simulink model "Lab_PMSM_Trial2"  (R2024a)
settings: Solver=VariableStepAuto  StartTime=0.0  StopTime=10  RelTol=1e-3
libraries: spsabctoAlphaBetaZeroLib x2
settings Model: Creator=VICTUS  LastModifiedBy=VICTUS

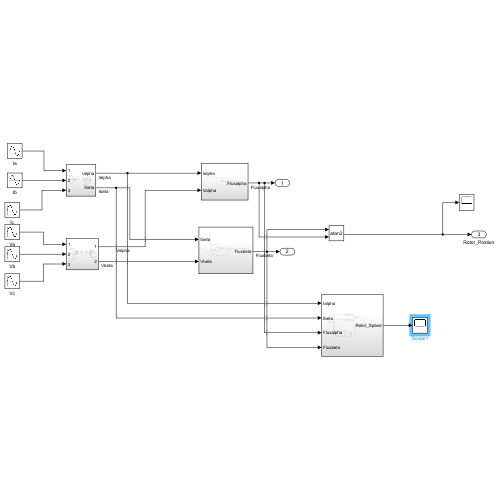
[thumbnail: Simulink's stored preview of the top-level diagram]
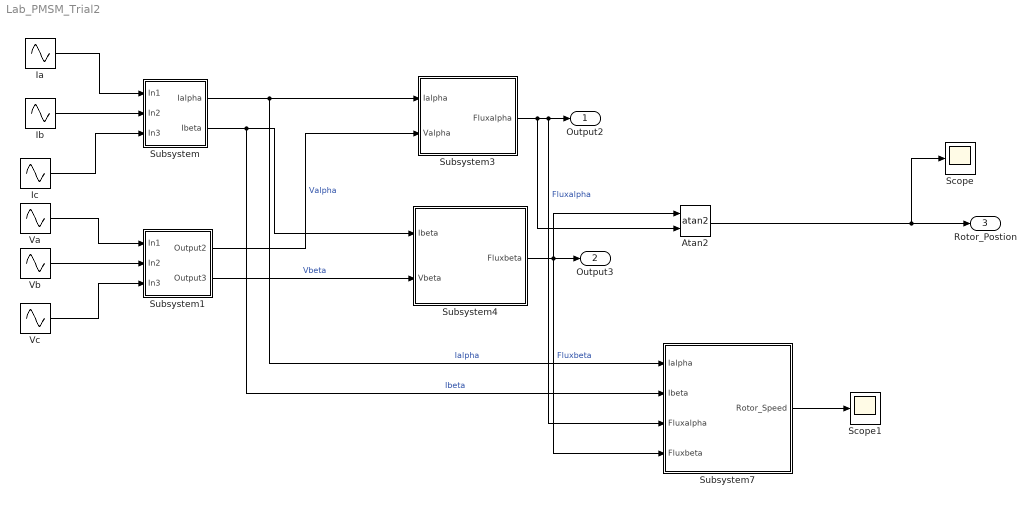
== system Lab_PMSM_Trial2 ==
  Atan2 : Trigonometry  Operator=atan2
  Ia : Sin  Amplitude=2  Frequency=300  SampleTime=0
  Ib : Sin  Amplitude=2  Frequency=300  Phase=-(120/180)*pi  SampleTime=0
  Ic : Sin  Amplitude=2  Frequency=300  Phase=(120/180)*pi  SampleTime=0
  Scope : Scope
  Scope1 : Scope
  Subsystem : Subsystem
  Subsystem1 : Subsystem
  Subsystem3 : Subsystem
  Subsystem4 : Subsystem
  Subsystem7 : Subsystem
  Va : Sin  Amplitude=12  Frequency=300  SampleTime=0
  Vb : Sin  Amplitude=12  Frequency=300  Phase=-(120/180)*pi  SampleTime=0
  Vc : Sin  Amplitude=12  Frequency=300  Phase=(120/180)*pi  SampleTime=0
  Output2 : Outport
  Output3 : Outport  Port=2
  Rotor_Postion : Outport  Port=3
  wires:
  Ic/1 -> Subsystem/3(In3)
  Ib/1 -> Subsystem/2(In2)
  Subsystem/1(Ialpha) -> Subsystem7/1(Ialpha), Subsystem3/1(Ialpha)  "Ialpha"
  Subsystem/2(Ibeta) -> Subsystem7/2(Ibeta), Subsystem4/1(Ibeta)  "Ibeta"
  Va/1 -> Subsystem1/1(In1)
  Vb/1 -> Subsystem1/2(In2)
  Vc/1 -> Subsystem1/3(In3)
  Subsystem1/1(Output2) -> Subsystem3/2(Valpha)  "Valpha"
  Subsystem1/2(Output3) -> Subsystem4/2(Vbeta)  "Vbeta"
  Ia/1 -> Subsystem/1(In1)
  Subsystem3/1(Fluxalpha) -> Atan2/2, Subsystem7/3(Fluxalpha), Output2/1  "Fluxalpha"
  Subsystem4/1(Fluxbeta) -> Subsystem7/4(Fluxbeta), Atan2/1, Output3/1  "Fluxbeta"
  Subsystem7/1(Rotor_Speed) -> Scope1/1
  Atan2/1 -> Scope/1, Rotor_Postion/1

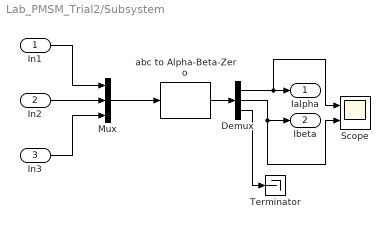
== system Lab_PMSM_Trial2/Subsystem ==
  In1 : Inport
  In2 : Inport  Port=2
  In3 : Inport  Port=3
  Demux : Demux  Outputs=3
  Mux : Mux  Inputs=3
  Scope : Scope  NumInputPorts=2
  Terminator : Terminator
  abc to Alpha-Beta-Zero : spsabctoAlphaBetaZeroLib/abc to Alpha-Beta-Zero
  Ialpha : Outport
  Ibeta : Outport  Port=2
  wires:
  Mux/1 -> abc to Alpha-Beta-Zero/1
  In1/1 -> Mux/1
  Demux/1 -> Scope/1, Ialpha/1
  abc to Alpha-Beta-Zero/1 -> Demux/1
  Demux/2 -> Scope/2, Ibeta/1
  In2/1 -> Mux/2
  In3/1 -> Mux/3
  Demux/3 -> Terminator/1

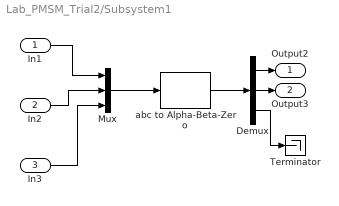
== system Lab_PMSM_Trial2/Subsystem1 ==
  In1 : Inport
  In2 : Inport  Port=2
  In3 : Inport  Port=3
  Demux : Demux  Outputs=3
  Mux : Mux  Inputs=3
  Terminator : Terminator
  abc to Alpha-Beta-Zero : spsabctoAlphaBetaZeroLib/abc to Alpha-Beta-Zero
  Output2 : Outport
  Output3 : Outport  Port=2
  wires:
  abc to Alpha-Beta-Zero/1 -> Demux/1
  In2/1 -> Mux/2
  Mux/1 -> abc to Alpha-Beta-Zero/1
  Demux/1 -> Output2/1
  Demux/2 -> Output3/1
  In3/1 -> Mux/3
  Demux/3 -> Terminator/1
  In1/1 -> Mux/1

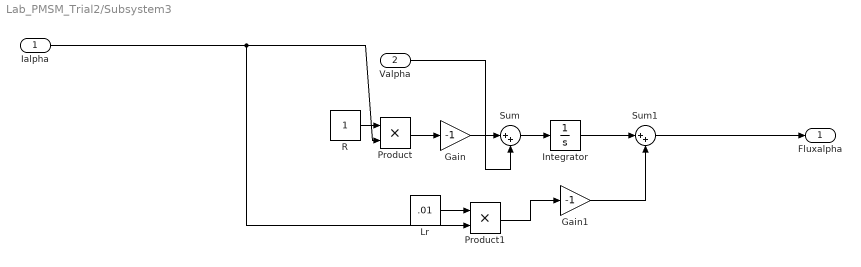
== system Lab_PMSM_Trial2/Subsystem3 ==
  Ialpha : Inport
  Valpha : Inport  Port=2
  Gain : Gain  Gain=-1
  Gain1 : Gain  Gain=-1
  Integrator : Integrator
  Lr : Constant  Value=.01
  Product : Product
  Product1 : Product
  R : Constant
  Sum : Sum  Inputs=|++
  Sum1 : Sum  Inputs=|++
  Fluxalpha : Outport
  wires:
  Sum/1 -> Integrator/1
  R/1 -> Product/1
  Integrator/1 -> Sum1/1
  Product/1 -> Gain/1
  Product1/1 -> Gain1/1
  Gain1/1 -> Sum1/2
  Lr/1 -> Product1/1
  Gain/1 -> Sum/1
  Ialpha/1 -> Product1/2, Product/2
  Sum1/1 -> Fluxalpha/1
  Valpha/1 -> Sum/2

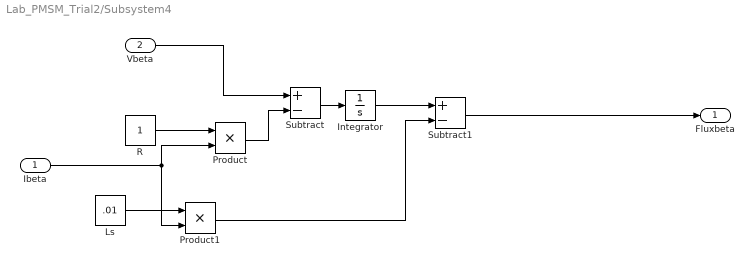
== system Lab_PMSM_Trial2/Subsystem4 ==
  Ibeta : Inport
  Vbeta : Inport  Port=2
  Integrator : Integrator
  Ls : Constant  Value=.01
  Product : Product
  Product1 : Product
  R : Constant
  Subtract : Sum  Inputs=+-
  Subtract1 : Sum  Inputs=+-
  Fluxbeta : Outport
  wires:
  Subtract/1 -> Integrator/1
  Product1/1 -> Subtract1/2
  Ibeta/1 -> Product/2, Product1/2
  Product/1 -> Subtract/2
  Integrator/1 -> Subtract1/1
  Ls/1 -> Product1/1
  R/1 -> Product/1
  Subtract1/1 -> Fluxbeta/1
  Vbeta/1 -> Subtract/1

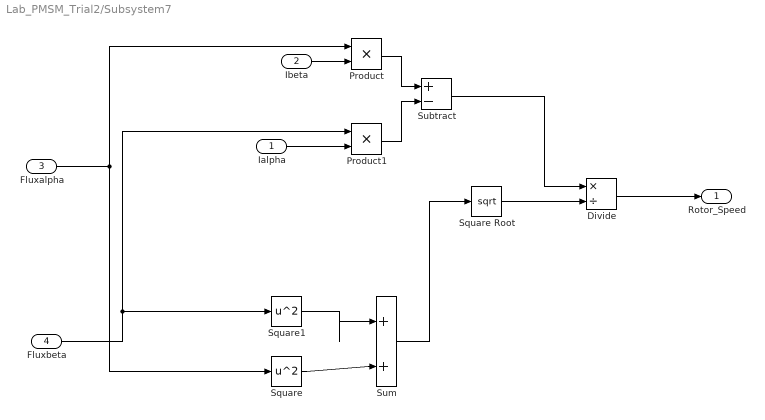
== system Lab_PMSM_Trial2/Subsystem7 ==
  Ialpha : Inport
  Ibeta : Inport  Port=2
  Fluxalpha : Inport  Port=3
  Fluxbeta : Inport  Port=4
  Divide : Product  Inputs=*/
  Product : Product
  Product1 : Product
  Square : Math  Operator=square
  Square Root : Sqrt
  Square1 : Math  Operator=square
  Subtract : Sum  Inputs=+-
  Sum : Sum  Inputs=|++
  Rotor_Speed : Outport
  wires:
  Product/1 -> Subtract/1
  Square/1 -> Sum/2
  Square1/1 -> Sum/1
  Divide/1 -> Rotor_Speed/1
  Ibeta/1 -> Product/2
  Square Root/1 -> Divide/2
  Subtract/1 -> Divide/1
  Fluxbeta/1 -> Product1/1, Square1/1
  Product1/1 -> Subtract/2
  Sum/1 -> Square Root/1
  Fluxalpha/1 -> Product/1, Square/1
  Ialpha/1 -> Product1/2
